simulink model "LAB_7"  (R2021a)
settings: Solver=VariableStepAuto  StartTime=0.0  StopTime=10.0  MaxStep=1e-3  RelTol=1e-3
settings Model: Creator=MAC  LastModifiedBy=MAC

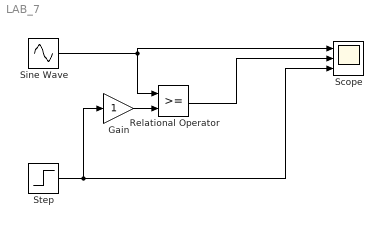
== system LAB_7 ==
  Gain : Gain
  Relational Operator : RelationalOperator  OutDataTypeStr=boolean  RndMeth=Simplest
  Scope : Scope  NumInputPorts=3
  Sine Wave : Sin  SampleTime=0
  Step : Step  Time=2  SampleTime=0
  wires:
  Sine Wave/1 -> Relational Operator/1, Scope/1
  Relational Operator/1 -> Scope/2
  Step/1 -> Gain/1, Scope/3
  Gain/1 -> Relational Operator/2
